simulink library "ThrustCurve_ul"  (R2020a)
settings: Solver=VariableStepAuto  StartTime=0.0  StopTime=10.0  RelTol=1e-3
undefined symbols (not defined in the file): Mot
settings Model: Creator=bunce  LastModifiedBy=bunce

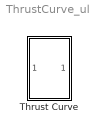
== system ThrustCurve_ul ==
  Thrust Curve : Subsystem

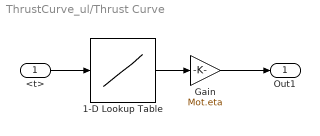
== system ThrustCurve_ul/Thrust Curve ==
  <t> : Inport
  1-D Lookup Table : Lookup_n-D  NumberOfTableDimensions=1  BreakpointsForDimension1=Mot.T_b  Table=Mot.F_th  InternalRulePriority=Speed  RndMeth=Simplest  InputSameDT=on
  Gain : Gain  Gain=Mot.eta
  Out1 : Outport
  wires:
  1-D Lookup Table/1 -> Gain/1
  Gain/1 -> Out1/1
  <t>/1 -> 1-D Lookup Table/1
